simulink model "Last_Model_Interior_team"  (R2017b)
settings: Solver=VariableStepAuto  SolverName=FixedStepDiscrete  StartTime=0.0  StopTime=10  FixedStep=1e-6
PreLoadFcn:
  | %% Motor Parameters
  | Rs=6.9*10^-3;
  | Ld=220*10^-6;
  | Lq=265.4*10^-6;
  | Pm=87.78*10^-3;
  | P=4;
  | b=0.0019;
  | J=0.13;
  | f=50;
  | P_Rated=100000;
  | N_Rated=6320;
  | N_max=30000;
  | Tfl=P_Rated/(N_Rated*(2*pi/60));
  | Tl=0;
  | 
  | %% hardware impl
  | Vdc=340;
  | clocking=100;
  | fs=10000;
  | Ts=1/fs;
  | Irated=500;
  | Imax=500;
  | Id_MAX=-(Pm/Ld);
  | I_Limit=Irated;
  | I_fw=I_Limit;
  | Vmax=Vdc/sqrt(3);
  | update=2;
  | 
  | 
  | %% Inverter
  | Vdc=340;
  | deadtime=1e-6;
  | 
  | 
  | 
  | %% Tuning OF Id_Pole_Placment
  | zeta_Id=0.707;
  | Gamma_Id=0.9;
  | Wn_Id=(1/(1-Gamma_Id))*(Rs/Ld);
  | Kc_Id=(2*zeta_Id*Ld*Wn_Id)-Rs;
  | TAW_Id=((2*zeta_Id*Wn_Id*Ld)-Rs)/(Ld*Wn_Id*Wn_Id);
  | 
  | %% Tuning OF Iq_Pole_Placment
  | zeta_Iq=0.707;
  | Gamma_Iq=0.9;
  | Wn_Iq=(1/(1-Gamma_Iq))*(Rs/Lq);
  | Kc_Iq=(2*zeta_Iq*Lq*Wn_Iq)-Rs;
  | TAW_Iq=((2*zeta_Iq*Wn_Iq*Lq)-Rs)/(Lq*Wn_Iq*Wn_Iq);
  | 
  | 
  | 
  | %% Tuning of PI Using Symmetric Optimum For q phase
  | Tc=(1/fs)/update;
  | A=8;
  | Kp_SO_q=Lq/(A*(Tc)*1.5);
  | Ki_SO_q=1/((A^2)*1.5*Tc);
  | %% Tuning of PI Using Symmetric Optimum For d phase
  | Kp_SO_d=Ld/(A*(Tc)*1.5);
  | Ki_SO_d=1/((A^2)*1.5*Tc);
  | 
  | 
  | %% Tuning Of PI Using Magnetuide Optimum Q_phase
  | Ki_MO_q=Rs/Lq;
  | Kp_MO_q=Lq/(2*1.5*Tc);
  | %% Tuning Of PI Using Magnetuide Optimum D_phase
  | Ki_MO_d=Rs/Ld;
  | Kp_MO_d=Ld/(2*1.5*Tc);
  | %% Tuning Parameter
  | Kp_d=Kp_MO_d;
  | Ki_d=Ki_MO_d;
  | Kp_q=Kp_MO_q;
  | Ki_q=Ki_MO_q;
  | 
  | 
  | 
  | %% Tuning Speed Loop
  | Tcc=Tc*10;
  | M=4;
  | Kp_Speed=(8*J)/(3*M*9*Pm*Tcc);
  | Ki_Speed=M*M*Tcc;
InitFcn:
  | %% Motor Parameters
  | Rs=6.9*10^-3;
  | Ld=220*10^-6;
  | Lq=265.4*10^-6;
  | Pm=87.78*10^-3;
  | P=4;
  | b=0.0019;
  | J=0.13;
  | f=50;
  | P_Rated=100000;
  | N_Rated=6320;
  | N_max=30000;
  | Tfl=P_Rated/(N_Rated*(2*pi/60));
  | Tl=0;
  | 
  | %% hardware impl
  | Vdc=340;
  | clocking=100;
  | fs=10000;
  | Ts=1/fs;
  | Irated=500;
  | Imax=500;
  | Id_MAX=-(Pm/Ld);
  | I_Limit=Irated;
  | I_fw=I_Limit;
  | Vmax=Vdc/sqrt(3);
  | update=2;
  | 
  | %% Inverter
  | Vdc=340;
  | deadtime=1e-6;
  | 
  | 
  | 
  | %% Tuning OF Id_Pole_Placment
  | zeta_Id=0.707;
  | Gamma_Id=0.9;
  | Wn_Id=(1/(1-Gamma_Id))*(Rs/Ld);
  | Kc_Id=(2*zeta_Id*Ld*Wn_Id)-Rs;
  | TAW_Id=((2*zeta_Id*Wn_Id*Ld)-Rs)/(Ld*Wn_Id*Wn_Id);
  | 
  | %% Tuning OF Iq_Pole_Placment
  | zeta_Iq=0.707;
  | Gamma_Iq=0.9;
  | Wn_Iq=(1/(1-Gamma_Iq))*(Rs/Lq);
  | Kc_Iq=(2*zeta_Iq*Lq*Wn_Iq)-Rs;
  | TAW_Iq=((2*zeta_Iq*Wn_Iq*Lq)-Rs)/(Lq*Wn_Iq*Wn_Iq);
  | 
  | 
  | 
  | %% Tuning of PI Using Symmetric Optimum For q phase
  | Tc=(1/fs)/update;
  | A=8;
  | Kp_SO_q=Lq/(A*(Tc)*1.5);
  | Ki_SO_q=1/((A^2)*1.5*Tc);
  | %% Tuning of PI Using Symmetric Optimum For d phase
  | Kp_SO_d=Ld/(A*(Tc)*1.5);
  | Ki_SO_d=1/((A^2)*1.5*Tc);
  | 
  | 
  | %% Tuning Of PI Using Magnetuide Optimum Q_phase
  | Ki_MO_q=Rs/Lq;
  | Kp_MO_q=Lq/(2*1.5*Tc);
  | %% Tuning Of PI Using Magnetuide Optimum D_phase
  | Ki_MO_d=Rs/Ld;
  | Kp_MO_d=Ld/(2*1.5*Tc);
  | %% Tuning Parameter
  | Kp_d=Kp_MO_d;
  | Ki_d=Ki_MO_d;
  | Kp_q=Kp_MO_q;
  | Ki_q=Ki_MO_q;
  | 
  | 
  | 
  | %% Tuning Speed Loop
  | Tcc=Tc*10;
  | M=4;
  | Kp_Speed=(8*J)/(3*M*9*Pm*Tcc);
  | Ki_Speed=M*M*Tcc;
undefined symbols (not defined in the file): DiscIntNeverNeededParam, magnitude
libraries: simulink x81, powerlib x14
(part 1 of 4)
CloseFcn:
  | clc;
  | clear;
settings Model: PauseTimes=0.2  Creator=oem  LastModifiedBy=Abdo
settings SolverCC: ZeroCrossAlgorithm=Adaptive
settings DataIOCC: SaveOutput=off  DSMLogging=off  SaveTime=off
settings OptimizationCC: UseDivisionForNetSlopeComputation=on  UseFloatMulNetSlope=on  DefaultUnderspecifiedDataType=single  EnhancedBackFolding=on  BooleansAsBitfields=on  PassReuseOutputArgsAs=Individual arguments  StateBitsets=on  DataBitsets=on  ZeroExternalMemoryAtStartup=off  ZeroInternalMemoryAtStartup=off  NoFixptDivByZeroProtection=on  EfficientFloat2IntCast=on  LifeSpan=1  MaxStackSize=64  OptimizeBlockOrder=speed  DifferentSizesBufferReuse=on
settings DebuggingCC: IgnoredZcDiagnostic=none  ParameterTunabilityLossMsg=error  UnconnectedInputMsg=none  UnconnectedOutputMsg=none  UnconnectedLineMsg=none
settings HardwareCC: ProdBitPerPointer=32  ProdBitPerSizeT=32  ProdBitPerPtrDiffT=32  ProdLargestAtomicFloat=None  ProdWordSize=32  ProdHWDeviceType=Atmel->AVR (32-bit)
settings ModelReferenceCC: EnableRefExpFcnMdlSchedulingChecks=off
settings SFSimCC: SimUseLocalCustomCode=on  MATLABDynamicMemAlloc=off
settings RTWCC: SystemTargetFile=ert.tlc  TemplateMakefile=ert_default_tmf  RTWUseLocalCustomCode=on  Toolchain=Texas Instruments Code Composer Studio (C2000)
settings CodeAppCC: ForceParamTrailComments=on  IgnoreCustomStorageClasses=off  OperatorAnnotations=on  SimulinkDataObjDesc=on  SFDataObjDesc=on  CustomSymbolStrGlobalVar=rt$N$M  CustomSymbolStrType=$N$M  CustomSymbolStrFcn=$N$M$F  CustomSymbolStrMacro=$N$M  InsertBlockDesc=on
settings ERTTargetCC: IncludeMdlTerminateFcn=off  CombineSignalStateStructs=on  CodeInterfacePackaging=Reusable function  SupportComplex=off  SupportNonInlinedSFcns=on  ExtModeStaticAlloc=on  ERTCustomFileTemplate=example_file_process.tlc  ERTFilePackagingFormat=CompactWithDataFile  MemSecPackage=Simulink

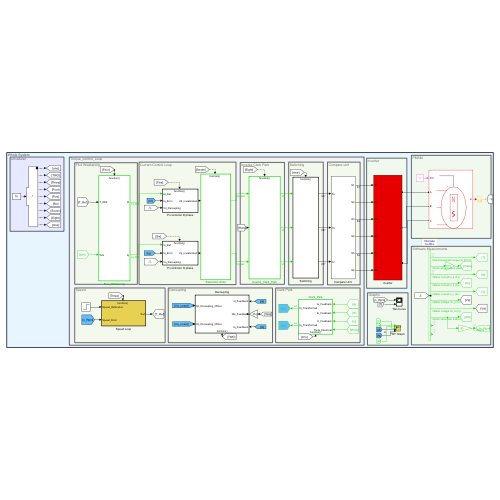
[thumbnail: Simulink's stored preview of the top-level diagram]
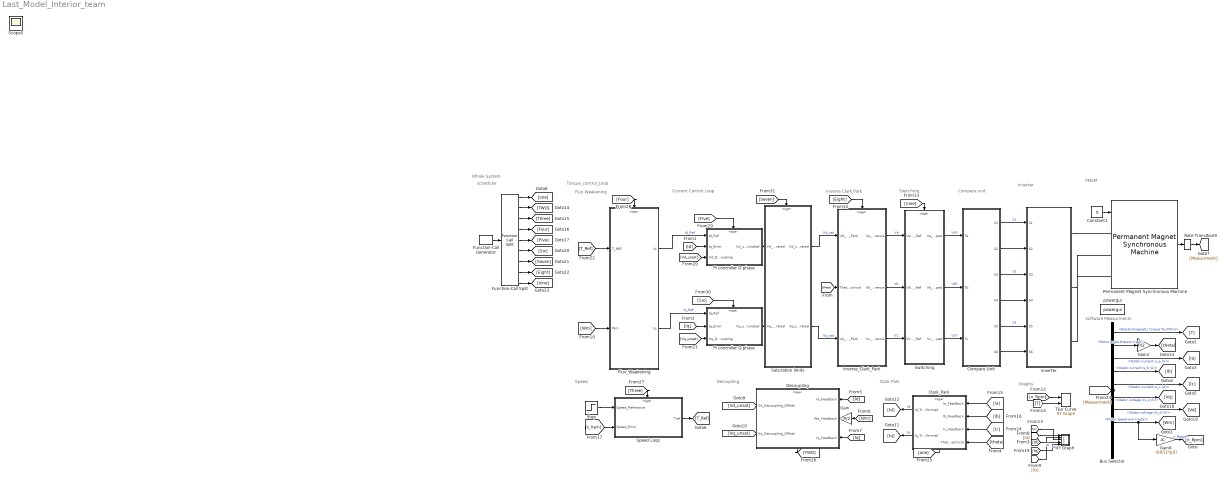
== system Last_Model_Interior_team ==
  note: schedular
  note: Software Measurments
  note: Torque_control_Loop
  note: Graphs
  note: Clark Park
  note: Flux Weakening
  note: Inverter
  note: Whole System
  note: Decoupling
  note: Inverse Clark Park
  note: Current Control Loop
  note: PMSM
  note: Switching
  note: Speed
  note: Compare unit
  Bus Selector : BusSelector  OutputSignals=Electromagnetic torque Te (N*m),Rotor angle thetam (rad),Stator current is_a (A),Stator current is_b (A),Stator current is_c (A),Stator voltage Vs_q (V),Stator voltage Vs_d (V),Rotor speed wm (rad/s),Stator current is_q (A),Stator current is_d (A)
  Clark_Park : Subsystem  TreatAsAtomicUnit=on
  "Compare Unit " : Subsystem
  Constant1 : Constant  Value=0
  Decoupling : Subsystem  TreatAsAtomicUnit=on
  Flux_Weakening : Subsystem
  Function-Call Generator : simulink/Ports & Subsystems/Function-Call Generator  sample_time=Tc  numberOfIterations=1
  Function-Call Split : FunctionCallSplit  IconShape=distinctive  NumOutputPorts=9  OutputPortLayout=default
  Gain : Gain  Gain=P/2
  Gain2 : Gain  Gain=P/2
  Gain8 : Gain  Gain=(60/(2*pi))
  Inverse_Clark_Park : Subsystem
  Permanent Magnet Synchronous Machine : powerlib/Machines/Permanent Magnet Synchronous Machine  NbPhases=3  FluxDistribution=Sinusoidal  RotorType=Salient-pole  MechanicalLoad=Torque Tm  PresetModel=No  ShowDetailedParameters=on  MeasurementBus=off  Resistance=Rs  Inductance=8.5e-3  dqInductances=[Ld Lq]  La=Ld  MachineConstant=Flux linkage established by magnets (V.s)  Flux=Pm  VoltageCst=31.8431  TorqueCst=0.26334  Flat=120  Mechanical=[J b P/2 0]  PolePairs=4  InitialConditions=[0,0, 0,0]  InitialConditions5ph=[0 0 0 0 0 0]  RefAngle=Aligned with phase A axis (original Park)  IterativeDiscreteModel=Trapezoidal non iterative  TsBlock=-1  TsPowergui=0
  Pi controller D phase : Subsystem
  Pi controller Q phase : Subsystem
  Rate Transition9 : RateTransition  OutPortSampleTime=Tc
  Saturation limits : Subsystem
  Speed Loop : Subsystem
  Step : Step  Time=0.000000001  After=5000  SampleTime=0
  Switching : Subsystem  SystemSampleTime=1e-4
  T&n Curve : simulink/Sinks/XY Graph  xmin=-1  xmax=1  ymin=-1  ymax=1  st=-1
  XY Graph : Subsystem  Description=Replaced Block  mask(Replaced Block){}
      mask help: This block has been replaced with an empty subsystem because it used functionality that is unavailable in Simulink R2017b.
      mask Display: fprintf('Replaced: %s\n','Record')
  inverter : Subsystem
  powergui : powerlib/powergui  Priority=1  SimulationMode=Discrete  SampleTime=1e-6  frequency=60  Iterations=50  frequencyindice=0  Pbase=100e6  ErrMax=1e-4  UnitsV=kV  UnitsW=MW  buscounter=0  FunctionMessages=off  echomessages=off  EnableUseOfTLC=off  CurrentSourceSwitches=off  DisableSnubberDevices=off  DisableRonSwitches=off  DisableVfSwitches=off  DisplayEquations=off  AutomaticDiscreteSolvers=off  SolverType=Tustin/Backward Euler (TBE)  Interpol=off  ExternalGateDelay=off  methode=off  Ts=100  x0status=blocks  SPID=on  SwTol=0  HookPort=off  NonlinearTolerance=1e-4  nMaxIteration=100  ContinueOnMaxIteration=off  RestoreLinks=warning  ResistiveCurrentMeasurement=off  Frange=[0:2:500]  Ylog=off  Xlog=on  ShowGrid=off  save=off  variable=ZData  structure=0  ZoomFFT=off  StartTime=0.0  cycles=1  DisplayStyle=1  fundamental=60  FreqAxis=off  MaxFrequency=1000  frequencyindicesteady=1  RmsSteady=1  display=off
  Scope5 : Scope
  wires:
  [Id] -> Decoupling/1(Id_Feedback)
  [Iq] -> Decoupling/3(Iq_Feedback)
  Decoupling/1(Vd_Decoupling_Offset) -> [Vd_unsat]
  Decoupling/2(Vq_Decoupling_Offset) -> [Vq_unsat]
  [Wm] -> Gain/1
  Gain/1 -> Decoupling/2(We_Feedback)
  [theta] -> Inverse_Clark_Park/2(Theta_Electrical)
  [n_Rpm] -> T&n Curve/1
  [T] -> T&n Curve/2
  [Ia] -> Clark_Park/1(Ia_Feedback)
  [Ib] -> Clark_Park/2(Ib_Feedback)
  [theta] -> Clark_Park/4(Theta_Electrical)
  Clark_Park/1(Id_Transformed) -> [Id]  "Id"
  Clark_Park/2(Iq_Transformed) -> [Iq]  "Iq"
  [Iq] -> XY Graph/5(In5)  "iq"
  [Id] -> XY Graph/4(In4)  "id"
  Saturation limits/1(Vd_saturated) -> Inverse_Clark_Park/1(Vd_Refrence_To_Inverse_Clark_Park)  "Vd_sat"
  Saturation limits/2(Vq_saturated) -> Inverse_Clark_Park/3(Vq_Refrence_To_Inverse_Clark_Park)  "Vq_sat"
  Bus Selector/1 -> [T]  "<Electromagnetic torque Te (N*m)>"
  Bus Selector/2 -> Gain2/1  "<Rotor angle thetam (rad)>"
  Bus Selector/4 -> [Ib]  "<Stator current is_b (A)>"
  Permanent Magnet Synchronous Machine/1 -> Rate Transition9/1
  Rate Transition9/1 -> [Measurment]
  Bus Selector/3 -> [Ia]  "<Stator current is_a (A)>"
  Bus Selector/5 -> [Ic]  "<Stator current is_c (A)>"
  Bus Selector/8 -> [Wm], Gain8/1  "<Rotor speed wm (rad/s)>"
  Gain8/1 -> [n_Rpm]  "n_Rpppm"
  [Wm] -> Flux_Weakening/2(Wm)
  Bus Selector/6 -> [Vq]  "<Stator voltage Vs_q (V)>"
  Bus Selector/7 -> [Vd]  "<Stator voltage Vs_d (V)>"
  Constant1/1 -> Permanent Magnet Synchronous Machine/1
  [Ia] -> XY Graph/1(In1)
  [Ib] -> XY Graph/2(In2)
  [Ic] -> XY Graph/3(In3)
  [Measurment] -> Bus Selector/1
  Inverse_Clark_Park/1(Va_Sin_Wave_Reference) -> Switching/1(Va_Sin_Ref)  "Va"
  Inverse_Clark_Park/2(Vb_Sin_Wave_Reference) -> Switching/2(Vb_Sin_Ref)  "Vb"
  Inverse_Clark_Park/3(Vc_Sin_Wave_Reference) -> Switching/3(Vc_Sin_Ref)  "VC"
  [Ic] -> Clark_Park/3(Ic_Feedback)
  [T_Ref] -> Flux_Weakening/1(T_REF)
  Switching/1(Va_Bus_Clamped) -> "Compare Unit "/1(Ta)  "VA*"
  Switching/2(Vb_Bus_Clamped) -> "Compare Unit "/2(Tb)  "VB*"
  Switching/3(Vc_Bus_Clamped) -> "Compare Unit "/3(Tc)  "VC*"
  "Compare Unit "/1(S1) -> inverter/1(S1)  "S1"
  "Compare Unit "/2(S2) -> inverter/2(S2)
  "Compare Unit "/4(S4) -> inverter/4(S4)
  "Compare Unit "/6(S6) -> inverter/6(S6)
  "Compare Unit "/3(S3) -> inverter/3(S3)  "S2"
  "Compare Unit "/5(S5) -> inverter/5(S5)  "S3"
  Step/1 -> Speed Loop/1(Speed_Referance)
  [n_Rpm] -> Speed Loop/2(Speed_Error)
  Speed Loop/1(Tref) -> [T_Ref]
  Flux_Weakening/1(Id) -> Pi controller D phase/1(Id_Ref)  "Id_Ref"
  [Id] -> Pi controller D phase/2(Iq_Error)
  [Vd_unsat] -> Pi controller D phase/3(Vd_Decoupling)
  Pi controller D phase/1(Vd_unsaturated) -> Saturation limits/1(Vd_unsaturated)
  Flux_Weakening/2(Iq) -> Pi controller Q phase/1(Iq_Ref)  "Iq_Ref"
  [Iq] -> Pi controller Q phase/2(Iq_Error)
  [Vq_unsat] -> Pi controller Q phase/3(Vq_Decoupling)
  Pi controller Q phase/1(Vq_unsaturated) -> Saturation limits/2(Vq_unsaturated)
  Function-Call Generator/1 -> Function-Call Split/1
  [one] -> Clark_Park/Trigger
  Function-Call Split/1 -> [one]
  Function-Call Split/2 -> [TWO]
  Function-Call Split/3 -> [Three]
  Function-Call Split/4 -> [Four]
  Function-Call Split/5 -> [Five]
  Function-Call Split/6 -> [Six]
  Function-Call Split/7 -> [Seven]
  [TWO] -> Decoupling/Trigger
  [Four] -> Flux_Weakening/Trigger
  [Five] -> Pi controller D phase/Trigger
  [Six] -> Pi controller Q phase/Trigger
  [Seven] -> Saturation limits/Trigger
  Function-Call Split/8 -> [Eight]
  Function-Call Split/9 -> [nine]
  [Eight] -> Inverse_Clark_Park/Trigger
  [nine] -> Switching/Trigger
  Gain2/1 -> [theta]
  [Three] -> Speed Loop/Trigger
  connections:
  inverter/RConn1 -- Permanent Magnet Synchronous Machine/LConn1
  inverter/RConn2 -- Permanent Magnet Synchronous Machine/LConn2
  inverter/RConn3 -- Permanent Magnet Synchronous Machine/LConn3

== system Last_Model_Interior_team/Clark_Park ==
  Ia_Feedback : Inport
  Ib_Feedback : Inport  Port=2
  Ic_Feedback : Inport  Port=3
  Theta_Electrical : Inport  Port=4
  function : TriggerPort  TriggerType=function-call  VariantControl=(inherit)
  Constant : Constant  Value=(2*pi)/3
  Constant1 : Constant  Value=(4*pi)/3
  Constant2 : Constant  Value=(2*pi)/3
  Constant3 : Constant  Value=(4*pi)/3
  Cos2 : Trigonometry  Operator=cos
  Cos3 : Trigonometry  Operator=cos
  Cos4 : Trigonometry  Operator=cos
  Cos5 : Trigonometry
  Cos6 : Trigonometry
  Cos7 : Trigonometry
  Gain8 : Gain  Gain=2/3
  Gain9 : Gain  Gain=-2/3
  Product{4..9} (6 alike) : Product
  Sum{4..5,7..8} (4 alike) : Sum  Inputs=-+
  Sum6 : Sum  Inputs=+++
  Sum9 : Sum  Inputs=+++
  Id_Transformed : Outport
  Iq_Transformed : Outport  Port=2
  wires:
  Theta_Electrical/1 -> Cos5/1, Sum7/2, Sum8/2, Sum4/2, Cos2/1, Sum5/2
  Sum4/1 -> Cos3/1
  Constant/1 -> Sum4/1
  Constant1/1 -> Sum5/1
  Sum5/1 -> Cos4/1
  Cos2/1 -> Product4/2
  Cos3/1 -> Product5/1
  Cos4/1 -> Product6/1
  Product5/1 -> Sum6/2
  Product4/1 -> Sum6/1
  Product6/1 -> Sum6/3
  Sum6/1 -> Gain8/1
  Gain8/1 -> Id_Transformed/1
  Sum8/1 -> Cos7/1
  Gain9/1 -> Iq_Transformed/1
  Product8/1 -> Sum9/2
  Product9/1 -> Sum9/3
  Product7/1 -> Sum9/1
  Constant3/1 -> Sum8/1
  Cos7/1 -> Product9/1
  Constant2/1 -> Sum7/1
  Sum7/1 -> Cos6/1
  Cos6/1 -> Product8/1
  Sum9/1 -> Gain9/1
  Cos5/1 -> Product7/2
  Ia_Feedback/1 -> [a]
  Ib_Feedback/1 -> [b]
  Ic_Feedback/1 -> [c]
  [a] -> Product4/1
  [b] -> Product5/2
  [c] -> Product6/2
  [a] -> Product7/1
  [b] -> Product8/2
  [c] -> Product9/2

== system Last_Model_Interior_team/Compare Unit  ==
  Ta : Inport
  Tb : Inport  Port=2
  Tc : Inport  Port=3
  AND{,1..5} (6 alike) : Logic  IconShape=distinctive  AllPortsSameDT=off  OutDataTypeStr=boolean
  Add : Sum  Inputs=+-
  Carrier Wave1 : simulink/Sources/Repeating Sequence  rep_seq_t=[0 0.5 1]/((fs))  rep_seq_y=[0 100 0]
  NOT : Logic  Operator=NOT  IconShape=distinctive  AllPortsSameDT=off  OutDataTypeStr=boolean
  NOT1 : Logic  Operator=NOT  IconShape=distinctive  AllPortsSameDT=off  OutDataTypeStr=boolean
  NOT3 : Logic  Operator=NOT  IconShape=distinctive  AllPortsSameDT=off  OutDataTypeStr=boolean
  Relational Operator : RelationalOperator  OutDataTypeStr=boolean  RndMeth=Ceiling
  Relational Operator1 : RelationalOperator  OutDataTypeStr=boolean  RndMeth=Ceiling
  Relational Operator2 : RelationalOperator  OutDataTypeStr=boolean  RndMeth=Ceiling
  Scope : Scope  NumInputPorts=2
  Scope1 : Scope  NumInputPorts=2
  Scope2 : Scope
  Unit Delay{,1..5} (6 alike) : UnitDelay  SampleTime=deadtime  HasFrameUpgradeWarning=on
  S1 : Outport  VectorParamsAs1DForOutWhenUnconnected=off
  S2 : Outport  Port=2  VectorParamsAs1DForOutWhenUnconnected=off
  S3 : Outport  Port=3  VectorParamsAs1DForOutWhenUnconnected=off
  S4 : Outport  Port=4  VectorParamsAs1DForOutWhenUnconnected=off
  S5 : Outport  Port=5  VectorParamsAs1DForOutWhenUnconnected=off
  S6 : Outport  Port=6  VectorParamsAs1DForOutWhenUnconnected=off
  wires:
  Ta/1 -> Relational Operator/1, Scope1/1
  Tc/1 -> Relational Operator2/1
  Tb/1 -> Relational Operator1/1
  Relational Operator/1 -> Add/1, NOT/1, Unit Delay/1, AND/1
  Unit Delay/1 -> AND/2
  AND/1 -> Scope/1, S1/1, Add/2
  NOT/1 -> Unit Delay1/1, AND1/1
  Unit Delay1/1 -> AND1/2
  AND1/1 -> S2/1, Scope/2
  Unit Delay3/1 -> AND3/2
  NOT3/1 -> Unit Delay3/1, AND3/1
  Unit Delay2/1 -> AND2/2
  Relational Operator1/1 -> AND2/1, Unit Delay2/1, NOT3/1
  AND2/1 -> S3/1
  AND3/1 -> S4/1
  Relational Operator2/1 -> NOT1/1, Unit Delay4/1, AND4/1
  Unit Delay4/1 -> AND4/2
  NOT1/1 -> Unit Delay5/1, AND5/1
  Unit Delay5/1 -> AND5/2
  AND4/1 -> S5/1
  AND5/1 -> S6/1
  Add/1 -> Scope2/1
  Carrier Wave1/1 -> Scope1/2, Relational Operator/2, Relational Operator2/2, Relational Operator1/2  "Carrier_Wave"

== system Last_Model_Interior_team/Decoupling ==
  Id_Feedback : Inport
  We_Feedback : Inport  Port=2
  Iq_Feedback : Inport  Port=3
  function : TriggerPort  TriggerType=function-call  VariantControl=(inherit)
  Add : Sum
  Constant : Constant  Value=Ld
  Constant1 : Constant  Value=Lq
  Constant2 : Constant  Value=Pm
  Product : Product
  Product1 : Product
  Product2 : Product  Inputs=3
  Vd_Decoupling_Offset : Outport
  Vq_Decoupling_Offset : Outport  Port=2
  wires:
  Constant1/1 -> Product2/1
  Iq_Feedback/1 -> Product2/3
  Product2/1 -> Vd_Decoupling_Offset/1
  Id_Feedback/1 -> Product/2
  Product/1 -> Add/1
  Constant2/1 -> Add/2
  Product1/1 -> Vq_Decoupling_Offset/1
  We_Feedback/1 -> Product1/2, Product2/2
  Add/1 -> Product1/1
  Constant/1 -> Product/1

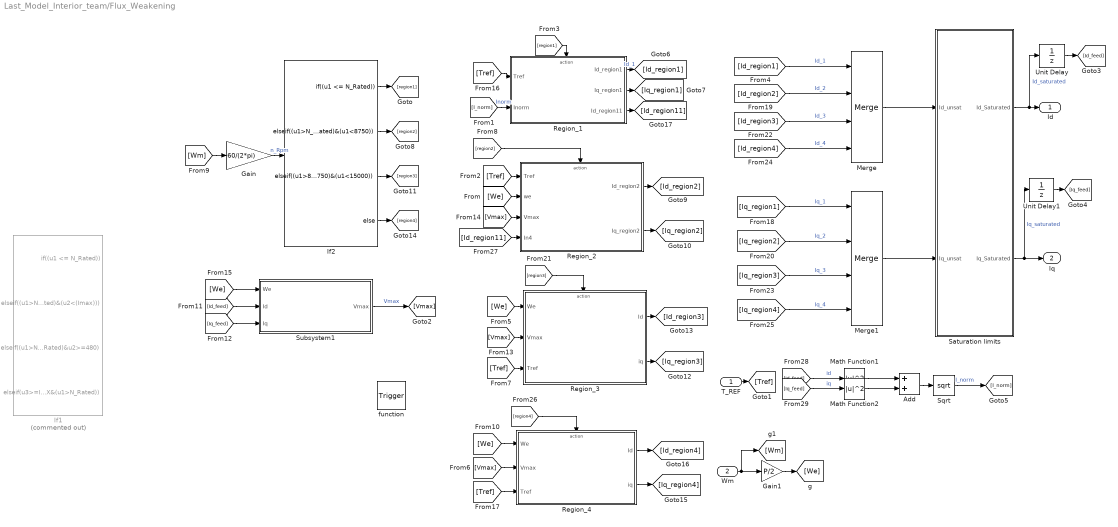
== system Last_Model_Interior_team/Flux_Weakening ==
  T_REF : Inport
  Wm : Inport  Port=2
  function : TriggerPort  TriggerType=function-call  VariantControl=(inherit)
  Add : Sum
  Gain : Gain  Gain=60/(2*pi)
  Gain1 : Gain  Gain=P/2
  If1 : If  Commented=on  NumInputs=3  IfExpression=(u1 <= N_Rated)  ElseIfExpressions=(u1>N_Rated)&(u2<(Imax)),(u1>N_Rated)&u2>=480,u3>=Id_MAX&(u1>N_Rated)  ShowElse=off
  If2 : If  IfExpression=(u1 <= N_Rated)  ElseIfExpressions=(u1>N_Rated)&(u1<8750),(u1>8750)&(u1<15000)
  Math Function1 : Math  Operator=magnitude^2  OutputSignalType=real  SaturateOnIntegerOverflow=on
  Math Function2 : Math  Operator=magnitude^2  OutputSignalType=real  SaturateOnIntegerOverflow=on
  Merge : Merge  Inputs=4
  Merge1 : Merge  Inputs=4
  Region_1 : Subsystem  TreatAsAtomicUnit=on
  Region_2 : Subsystem  TreatAsAtomicUnit=on
  Region_3 : Subsystem  TreatAsAtomicUnit=on
  Region_4 : Subsystem  TreatAsAtomicUnit=on
  Saturation limits : Subsystem
  Sqrt : Sqrt  OutputSignalType=real  SaturateOnIntegerOverflow=on
  Subsystem1 : Subsystem
  Unit Delay : UnitDelay  SampleTime=-1  HasFrameUpgradeWarning=on
  Unit Delay1 : UnitDelay  SampleTime=-1  HasFrameUpgradeWarning=on
  Id : Outport
  Iq : Outport  Port=2
  wires:
  [Tref] -> Region_1/1(Tref)
  Gain/1 -> If2/1  "n_Rpm"
  Wm/1 -> Gain1/1, [Wm]
  T_REF/1 -> [Tref]
  Gain1/1 -> [We]
  [Tref] -> Region_2/1(Tref)
  [We] -> Region_2/2(we)
  Sqrt/1 -> [I_norm]  "I_norm"
  [Id_feed] -> Math Function1/1  "id"
  Math Function1/1 -> Add/1
  Math Function2/1 -> Add/2
  Add/1 -> Sqrt/1
  [We] -> Region_3/1(We)
  [Iq_feed] -> Math Function2/1  "iq"
  [Id_feed] -> Subsystem1/2(Id)
  [We] -> Subsystem1/1(We)
  [Iq_feed] -> Subsystem1/3(Iq)
  Subsystem1/1(Vmax) -> [Vmax]  "Vmax"
  [Wm] -> Gain/1
  [Vmax] -> Region_2/3(Vmax)
  [Vmax] -> Region_3/2(Vmax)
  [I_norm] -> Region_1/2(Inorm)  "Inorm"
  [Vmax] -> Region_4/2(Vmax)
  [We] -> Region_4/1(We)
  Merge/1 -> Saturation limits/1(Id_unsat)
  Merge1/1 -> Saturation limits/2(Iq_unsat)
  Saturation limits/1(Id_Saturated) -> Unit Delay/1, Id/1  "Id_saturated"
  Saturation limits/2(Iq_Saturated) -> Iq/1, Unit Delay1/1  "Iq_saturated"
  [region1] -> Region_1/Action
  Region_1/1(Id_region1) -> [Id_region1]  "Id_1"
  Region_1/2(Iq_region1) -> [Iq_region1]
  [Id_region1] -> Merge/1  "Id_1"
  [Iq_region1] -> Merge1/1  "Iq_1"
  [region2] -> Region_2/Action
  Region_2/1(Id_region2) -> [Id_region2]
  Region_2/2(Iq_region2) -> [Iq_region2]
  [Id_region2] -> Merge/2  "Id_2"
  [Iq_region2] -> Merge1/2  "Iq_2"
  [region3] -> Region_3/Action
  Region_3/1(Id) -> [Id_region3]
  Region_3/2(iq) -> [Iq_region3]
  [Id_region3] -> Merge/3  "Id_3"
  [Iq_region3] -> Merge1/3  "Iq_3"
  Region_4/1(Id) -> [Id_region4]
  Region_4/2(iq) -> [Iq_region4]
  [Id_region4] -> Merge/4  "Id_4"
  [Iq_region4] -> Merge1/4  "Iq_4"
  [region4] -> Region_4/Action
  [Id_region11] -> Region_2/4(In4)
  Region_1/3(Id_region11) -> [Id_region11]
  If2/1 -> [region1]
  If2/2 -> [region2]
  If2/3 -> [region3]
  If2/4 -> [region4]
  [Tref] -> Region_3/3(Tref)
  [Tref] -> Region_4/3(Tref)
  Unit Delay/1 -> [Id_feed]
  Unit Delay1/1 -> [Iq_feed]

== system Last_Model_Interior_team/Inverse_Clark_Park ==
  Vd_Refrence_To_Inverse_Clark_Park : Inport
  Theta_Electrical : Inport  Port=2
  Vq_Refrence_To_Inverse_Clark_Park : Inport  Port=3
  function : TriggerPort  TriggerType=function-call  VariantControl=(inherit)
  Constant{1..4} (4 alike) : Constant  Value=(2*pi)/3
  Cos1 : Trigonometry  Operator=cos
  Cos2 : Trigonometry  Operator=cos
  Cos3 : Trigonometry
  Cos4 : Trigonometry
  Cos5 : Trigonometry  Operator=cos
  Cos6 : Trigonometry
  Gain : Gain  Gain=-1
  Gain1 : Gain  Gain=-1
  Gain2 : Gain  Gain=-1
  Product{1..2,4..5,7..8} (6 alike) : Product
  Sum{1..3,7,10} (5 alike) : Sum
  Sum5 : Sum  Inputs=-+
  Sum8 : Sum  Inputs=-+
  Va_Sin_Wave_Reference : Outport
  Vb_Sin_Wave_Reference : Outport  Port=2
  Vc_Sin_Wave_Reference : Outport  Port=3
  wires:
  Product4/1 -> Sum7/1
  Cos5/1 -> Product7/2
  Sum8/1 -> Cos6/1
  Product7/1 -> Sum10/1
  Cos6/1 -> Gain1/1
  Cos2/1 -> Product4/2
  Product8/1 -> Sum10/2
  Sum7/1 -> Va_Sin_Wave_Reference/1
  Sum10/1 -> Vb_Sin_Wave_Reference/1
  [d] -> Product7/1
  [d] -> Product4/1
  Constant2/1 -> Sum8/1
  [q] -> Product8/2
  Vd_Refrence_To_Inverse_Clark_Park/1 -> [d]
  Vq_Refrence_To_Inverse_Clark_Park/1 -> [q]
  [q] -> Product5/1
  Cos3/1 -> Gain/1
  Product5/1 -> Sum7/2
  Gain/1 -> Product5/2
  Constant1/1 -> Sum5/1
  Sum5/1 -> Cos5/1
  Gain1/1 -> Product8/1
  Gain2/1 -> Product2/1
  Sum2/1 -> Cos1/1
  Constant4/1 -> Sum2/1
  Theta_Electrical/1 -> Sum3/2, Sum2/2, Sum8/2, Sum5/2, Cos2/1, Cos3/1
  [q] -> Product2/2
  Constant3/1 -> Sum3/1
  [d] -> Product1/1
  Sum1/1 -> Vc_Sin_Wave_Reference/1
  Product2/1 -> Sum1/2
  Cos4/1 -> Gain2/1
  Product1/1 -> Sum1/1
  Sum3/1 -> Cos4/1
  Cos1/1 -> Product1/2

== system Last_Model_Interior_team/Pi controller D phase ==
  Id_Ref : Inport
  Iq_Error : Inport  Port=2
  Vd_Decoupling : Inport  Port=3
  function : TriggerPort  TriggerType=function-call  VariantControl=(inherit)
  Pi D Phase : Subsystem  TreatAsAtomicUnit=on
  Sum : Sum  Inputs=|+-
  Sum4 : Sum  Inputs=|+-
  Vd_unsaturated : Outport
  wires:
  Sum/1 -> Pi D Phase/1(Id*)  "error_Id"
  Iq_Error/1 -> Sum/2
  Pi D Phase/1(Vd) -> Sum4/1
  Id_Ref/1 -> Sum/1
  Sum4/1 -> Vd_unsaturated/1  "Vd_unsat"
  Vd_Decoupling/1 -> Sum4/2

== system Last_Model_Interior_team/Pi controller Q phase ==
  Iq_Ref : Inport
  Iq_Error : Inport  Port=2
  Vq_Decoupling : Inport  Port=3
  function : TriggerPort  TriggerType=function-call  VariantControl=(inherit)
  PI controller : Subsystem  TreatAsAtomicUnit=on
  Sum1 : Sum  Inputs=|+-
  Sum5 : Sum  Inputs=|++
  Vq_unsaturated : Outport
  wires:
  PI controller/1(Vq) -> Sum5/1
  Sum5/1 -> Vq_unsaturated/1  "Vq_unsat"
  Sum1/1 -> PI controller/1(Iq*)  "error_iq"
  Iq_Ref/1 -> Sum1/1
  Iq_Error/1 -> Sum1/2
  Vq_Decoupling/1 -> Sum5/2

== system Last_Model_Interior_team/Saturation limits ==
  Vd_unsaturated : Inport
  Vq_unsaturated : Inport  Port=2
  function : TriggerPort  TriggerType=function-call  VariantControl=(inherit)
  Abs : Abs
  Abs1 : Abs
  Add : Sum
  Constant : Constant  Value=Vmax
  Constant2 : Constant  Value=Vmax
  Divide : Product  Inputs=**/
  Divide1 : Product  Inputs=**/
  Math Function : Math  Operator=magnitude^2  SaturateOnIntegerOverflow=on
  Math Function1 : Math  Operator=magnitude^2  SaturateOnIntegerOverflow=on
  Multiply : Gain  Gain=-1
  Multiply1 : Gain  Gain=-1
  Saturation Dynamic : simulink/Discontinuities/Saturation Dynamic  OutMin=[]  OutMax=[]  OutDataTypeStr=Inherit: Same as second input  OutDataType=fixdt(1, 16)  OutScaling=2^-10  DoSatur=off
  Saturation Dynamic1 : simulink/Discontinuities/Saturation Dynamic  OutMin=[]  OutMax=[]  OutDataTypeStr=Inherit: Same as second input  OutDataType=fixdt(1, 16)  OutScaling=2^-10  DoSatur=off
  Sqrt : Sqrt  SaturateOnIntegerOverflow=on
  Zero detection : Subsystem
  Vd_saturated : Outport
  Vq_saturated : Outport  Port=2
  wires:
  Vd_unsaturated/1 -> [Vd_unsat], Abs1/1, Math Function1/1
  Math Function/1 -> Add/1
  Math Function1/1 -> Add/2
  Add/1 -> Sqrt/1
  Sqrt/1 -> Zero detection/1(In1)
  Zero detection/1(Out1) -> Divide1/3, Divide/3  "Vs_unsat"
  Vq_unsaturated/1 -> [Vq_unsat], Abs/1, Math Function/1
  Abs/1 -> Divide/2
  Constant/1 -> Divide/1
  Constant2/1 -> Divide1/1
  Abs1/1 -> Divide1/2
  Divide/1 -> Saturation Dynamic/1, Multiply/1
  [Vq_unsat] -> Saturation Dynamic/2
  Multiply/1 -> Saturation Dynamic/3
  [Vd_unsat] -> Saturation Dynamic1/2
  Divide1/1 -> Multiply1/1, Saturation Dynamic1/1
  Multiply1/1 -> Saturation Dynamic1/3
  Saturation Dynamic/1 -> Vq_saturated/1
  Saturation Dynamic1/1 -> Vd_saturated/1

== system Last_Model_Interior_team/Speed Loop ==
  Speed_Referance : Inport
  Speed_Error : Inport  Port=2
  function : TriggerPort  TriggerType=function-call  VariantControl=(inherit)
  Sum2 : Sum  Inputs=|+-
  speed_controller : Subsystem  TreatAsAtomicUnit=on
  Tref : Outport
  wires:
  Speed_Referance/1 -> Sum2/1
  Sum2/1 -> speed_controller/1(ref_speed)  "error_n"
  Speed_Error/1 -> Sum2/2
  speed_controller/1(T_ref) -> Tref/1

== system Last_Model_Interior_team/Switching ==
  Va_Sin_Ref : Inport
  Vb_Sin_Ref : Inport  Port=2
  Vc_Sin_Ref : Inport  Port=3
  function : TriggerPort  TriggerType=function-call  VariantControl=(inherit)
  +120_deg_Dpwm : Subsystem  Commented=on
  -120_deg_Dpwm : Subsystem  Commented=on
  30_deg_Dpwm : Subsystem  Commented=on
  60deg_+30_shifted : Subsystem  Commented=on
  60deg_-30_shifted : Subsystem  Commented=on
  60deg_DPWM : Subsystem
  SVpwm : Subsystem  Commented=on
  Scope : Scope  Commented=on  NumInputPorts=3
  Va_Bus_Clamped : Outport
  Vb_Bus_Clamped : Outport  Port=2
  Vc_Bus_Clamped : Outport  Port=3
  wires:
  ? -> +120_deg_Dpwm/2(Vb)
  ? -> +120_deg_Dpwm/3(Vc)
  ? -> +120_deg_Dpwm/1(Va)
  +120_deg_Dpwm/1(Va*) -> ?
  +120_deg_Dpwm/2(Vb*) -> ?
  +120_deg_Dpwm/3(Vc*) -> ?
  ? -> 30_deg_Dpwm/1(Va), Scope/1
  ? -> 30_deg_Dpwm/2(Vb), Scope/2
  ? -> 30_deg_Dpwm/3(Vc), Scope/3
  30_deg_Dpwm/3(Vc*) -> ?
  30_deg_Dpwm/2(Vb*) -> ?
  30_deg_Dpwm/1(Va*) -> ?
  Va_Sin_Ref/1 -> 60deg_DPWM/1(Va)
  Vb_Sin_Ref/1 -> 60deg_DPWM/2(Vb)
  Vc_Sin_Ref/1 -> 60deg_DPWM/3(Vc)
  60deg_DPWM/1(Va_Bus_Clamped) -> Va_Bus_Clamped/1
  60deg_DPWM/2(Vb_Bus_Clamped) -> Vb_Bus_Clamped/1
  60deg_DPWM/3(Vc_Bus_Clamped) -> Vc_Bus_Clamped/1

== system Last_Model_Interior_team/XY Graph ==
  In1 : Inport
  In2 : Inport  Port=2
  In3 : Inport  Port=3
  In4 : Inport  Port=4
  In5 : Inport  Port=5
  Terminator{1..5} (5 alike) : Terminator
  wires:
  In5/1 -> Terminator5/1
  In4/1 -> Terminator4/1
  In3/1 -> Terminator3/1
  In2/1 -> Terminator2/1
  In1/1 -> Terminator1/1

== system Last_Model_Interior_team/inverter ==
  S1 : Inport
  S2 : Inport  Port=2
  S3 : Inport  Port=3
  S4 : Inport  Port=4
  S5 : Inport  Port=5
  S6 : Inport  Port=6
  Current Measurement : powerlib/Measurements/Current Measurement  PhasorSimulation=off  OutputType=Complex  PSBequivalent=0
  DC Voltage Source : powerlib/Electrical Sources/DC Voltage Source  Amplitude=Vdc  Measurements=None
  IGBT/Diode : powerlib/Power Electronics/IGBT//Diode  Ron=1e-3  Rs=1e5  Cs=10e2  Measurements=on
  IGBT/Diode{1..5} (5 alike) : powerlib/Power Electronics/IGBT//Diode  Ron=1e-3  Rs=1e5  Cs=inf  Measurements=on
  Scope : Scope
  Scope2 : Scope
  Voltage Measurement : powerlib/Measurements/Voltage Measurement  PhasorSimulation=off  OutputType=Complex  PSBequivalent=0
  a : PMIOPort  Side=Right
  b : PMIOPort  Port=2  Side=Right
  c : PMIOPort  Port=3  Side=Right
  wires:
  S1/1 -> IGBT/Diode/1
  S2/1 -> IGBT/Diode1/1
  S3/1 -> IGBT/Diode2/1
  S4/1 -> IGBT/Diode3/1
  S5/1 -> IGBT/Diode4/1
  S6/1 -> IGBT/Diode5/1
  Current Measurement/1 -> Scope/1
  Voltage Measurement/1 -> Scope2/1
  connections:
  IGBT/Diode/LConn1 -- Current Measurement/RConn1 -- IGBT/Diode4/LConn1 -- IGBT/Diode2/LConn1
  IGBT/Diode5/LConn1 -- IGBT/Diode4/RConn1 -- c/RConn1
  IGBT/Diode3/RConn1 -- IGBT/Diode5/RConn1 -- Voltage Measurement/LConn2 -- DC Voltage Source/LConn1 -- IGBT/Diode1/RConn1
  IGBT/Diode2/RConn1 -- IGBT/Diode3/LConn1 -- b/RConn1
  IGBT/Diode1/LConn1 -- a/RConn1 -- IGBT/Diode/RConn1
  Voltage Measurement/LConn1 -- Current Measurement/LConn1 -- DC Voltage Source/RConn1

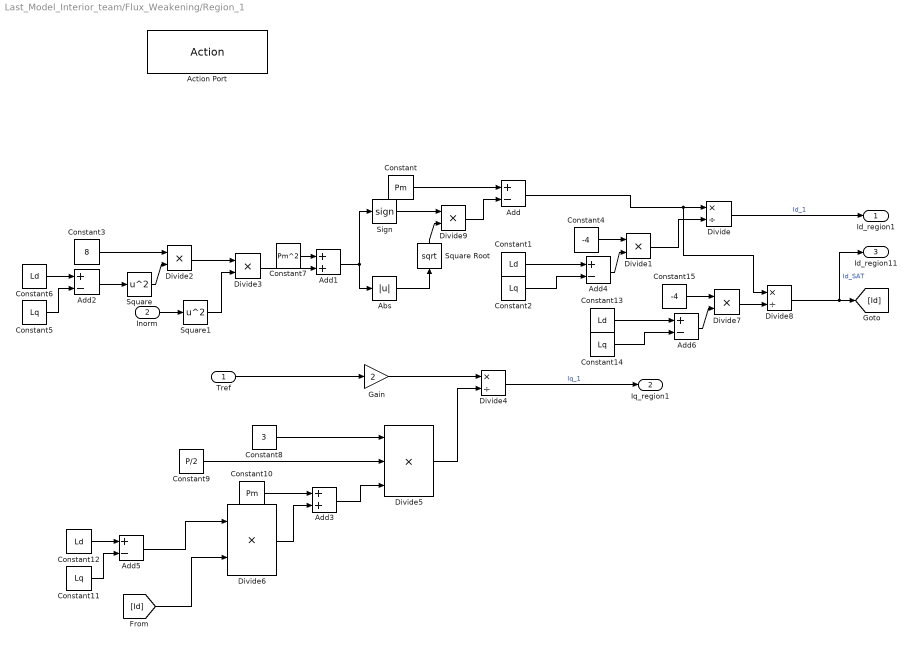
== system Last_Model_Interior_team/Flux_Weakening/Region_1 ==
  Tref : Inport
  Inorm : Inport  Port=2
  Action Port : ActionPort
  Abs : Abs
  Add{,2,4..6} (5 alike) : Sum  Inputs=+-
  Add1 : Sum
  Add3 : Sum
  Constant : Constant  Value=Pm
  Constant{1,6,12..13} (4 alike) : Constant  Value=Ld
  Constant10 : Constant  Value=Pm
  Constant{2,5,11,14} (4 alike) : Constant  Value=Lq
  Constant15 : Constant  Value=-4
  Constant3 : Constant  Value=8
  Constant4 : Constant  Value=-4
  Constant7 : Constant  Value=Pm^2
  Constant8 : Constant  Value=3
  Constant9 : Constant  Value=P/2
  Divide : Product  Inputs=*/
  Divide{1..3,6..7,9} (6 alike) : Product  Inputs=**
  Divide4 : Product  Inputs=*/
  Divide5 : Product  Inputs=***
  Divide8 : Product  Inputs=*/
  Gain : Gain  Gain=2
  Sign : Signum
  Square : Math  Operator=square  SaturateOnIntegerOverflow=on
  Square Root : Sqrt  SaturateOnIntegerOverflow=on
  Square1 : Math  Operator=square  SaturateOnIntegerOverflow=on
  Id_region1 : Outport  InitialOutput=[0]
  Iq_region1 : Outport  Port=2
  Id_region11 : Outport  Port=3  InitialOutput=[0]
  wires:
  Divide/1 -> Id_region1/1  "Id_1"
  Constant/1 -> Add/1
  Constant3/1 -> Divide2/1
  Add2/1 -> Square/1
  Constant5/1 -> Add2/2
  Constant6/1 -> Add2/1
  Square/1 -> Divide2/2
  Inorm/1 -> Square1/1
  Divide2/1 -> Divide3/1
  Square1/1 -> Divide3/2
  Abs/1 -> Square Root/1
  Add/1 -> Divide8/1, Divide/1
  Constant4/1 -> Divide1/1
  Constant1/1 -> Add4/1
  Constant2/1 -> Add4/2
  Add4/1 -> Divide1/2
  Divide1/1 -> Divide/2
  Divide3/1 -> Add1/2
  Constant7/1 -> Add1/1
  Add1/1 -> Sign/1, Abs/1
  Tref/1 -> Gain/1
  Gain/1 -> Divide4/1
  Constant8/1 -> Divide5/1
  Constant9/1 -> Divide5/2
  Constant10/1 -> Add3/1
  Constant12/1 -> Add5/1
  Constant11/1 -> Add5/2
  Add5/1 -> Divide6/1
  [Id] -> Divide6/2
  Divide6/1 -> Add3/2
  Add3/1 -> Divide5/3
  Divide5/1 -> Divide4/2
  Divide4/1 -> Iq_region1/1  "Iq_1"
  Add6/1 -> Divide7/2
  Constant14/1 -> Add6/2
  Constant13/1 -> Add6/1
  Constant15/1 -> Divide7/1
  Divide7/1 -> Divide8/2
  Divide8/1 -> Id_region11/1, [Id]  "Id_SAT"
  Square Root/1 -> Divide9/2
  Sign/1 -> Divide9/1
  Divide9/1 -> Add/2

== system Last_Model_Interior_team/Flux_Weakening/Region_2 ==
  Tref : Inport
  we : Inport  Port=2
  Vmax : Inport  Port=3
  In4 : Inport  Port=4
  Action Port : ActionPort
  Add3 : Sum
  Add5 : Sum  Inputs=+-
  Constant : Constant  Value=-500
  Constant1 : Constant  Value=-500
  Constant10 : Constant  Value=Pm
  Constant11 : Constant  Value=Lq
  Constant12 : Constant  Value=Ld
  Constant8 : Constant  Value=3
  Constant9 : Constant  Value=P/2
  Divide4 : Product  Inputs=*/
  Divide5 : Product  Inputs=***
  Divide6 : Product  Inputs=**
  Gain : Gain  Gain=2
  Saturation Dynamic : simulink/Discontinuities/Saturation Dynamic  OutMin=[]  OutMax=[]  OutDataTypeStr=Inherit: Same as second input  OutDataType=fixdt(1, 16)  OutScaling=2^-10  DoSatur=off
  Saturation Dynamic1 : simulink/Discontinuities/Saturation Dynamic  OutMin=[]  OutMax=[]  OutDataTypeStr=Inherit: Same as second input  OutDataType=fixdt(1, 16)  OutScaling=2^-10  DoSatur=off
  Subsystem : Subsystem
  Id_region2 : Outport
  Iq_region2 : Outport  Port=2
  wires:
  we/1 -> Subsystem/1(we)
  Vmax/1 -> Subsystem/3(Vmax)
  Subsystem/1(Id) -> Saturation Dynamic1/2, Saturation Dynamic/2
  Gain/1 -> Divide4/1
  Divide6/1 -> Add3/2
  Constant10/1 -> Add3/1
  Add5/1 -> Divide6/1
  Divide4/1 -> Iq_region2/1  "Iq_2"
  Add3/1 -> Divide5/3
  Constant9/1 -> Divide5/2
  Constant11/1 -> Add5/2
  Divide5/1 -> Divide4/2
  Constant8/1 -> Divide5/1
  Constant12/1 -> Add5/1
  [Id] -> Divide6/2
  Tref/1 -> Gain/1, Subsystem/2(Tref)
  Constant/1 -> Saturation Dynamic/3
  Saturation Dynamic/1 -> Id_region2/1  "Id_2"
  Constant1/1 -> Saturation Dynamic1/3
  In4/1 -> Saturation Dynamic1/1, Saturation Dynamic/1
  Saturation Dynamic1/1 -> [Id]  "Id_2"

== system Last_Model_Interior_team/Flux_Weakening/Region_3 ==
  We : Inport
  Vmax : Inport  Port=2
  Tref : Inport  Port=3
  Action Port : ActionPort
  Abs : Abs
  Add : Sum  Inputs=+-
  Add3 : Sum
  Add5 : Sum  Inputs=+-
  Constant : Constant  Value=I_Limit
  Constant10 : Constant  Value=Pm
  Constant11 : Constant  Value=Lq
  Constant12 : Constant  Value=Ld
  Constant8 : Constant  Value=3
  Constant9 : Constant  Value=P/2
  Divide4 : Product  Inputs=*/
  Divide5 : Product  Inputs=***
  Divide6 : Product  Inputs=**
  Gain : Gain  Gain=2
  Math Function1 : Math  Operator=magnitude^2  OutputSignalType=real  SaturateOnIntegerOverflow=on
  Math Function2 : Math  Operator=magnitude^2  OutputSignalType=real  SaturateOnIntegerOverflow=on
  Relational Operator : RelationalOperator  Operator=<=  OutDataTypeStr=boolean  RndMeth=Simplest
  Saturation : Saturate  UpperLimit=400  LowerLimit=-400
  Saturation1 : Saturate  UpperLimit=400  LowerLimit=-400
  Scope : Scope
  Sqrt : Sqrt  OutputSignalType=real  SaturateOnIntegerOverflow=on
  Subsystem1 : Subsystem
  Switch : Switch  Criteria=u2 > Threshold
  Id : Outport
  iq : Outport  Port=2
  wires:
  We/1 -> Subsystem1/1(We)
  Constant/1 -> Math Function2/1
  Math Function2/1 -> Add/1
  Math Function1/1 -> Add/2
  Add/1 -> Abs/1
  Sqrt/1 -> Switch/3, Relational Operator/2  "Iq_3"
  Vmax/1 -> Subsystem1/2(Vmax)
  Subsystem1/1(Id) -> [Id], Scope/1, Saturation1/1, Saturation/1  "Id_3"
  Abs/1 -> Sqrt/1
  Saturation/1 -> Math Function1/1
  Saturation1/1 -> Id/1  "Id_3"
  Divide6/1 -> Add3/2
  [Id] -> Divide6/2
  Add5/1 -> Divide6/1
  Constant8/1 -> Divide5/1
  Gain/1 -> Divide4/1
  Divide5/1 -> Divide4/2
  Constant12/1 -> Add5/1
  Constant10/1 -> Add3/1
  Add3/1 -> Divide5/3
  Constant9/1 -> Divide5/2
  Tref/1 -> Gain/1
  Constant11/1 -> Add5/2
  Divide4/1 -> Switch/1, Relational Operator/1  "Iq_3"
  Switch/1 -> iq/1  "Iq_3"
  Relational Operator/1 -> Switch/2

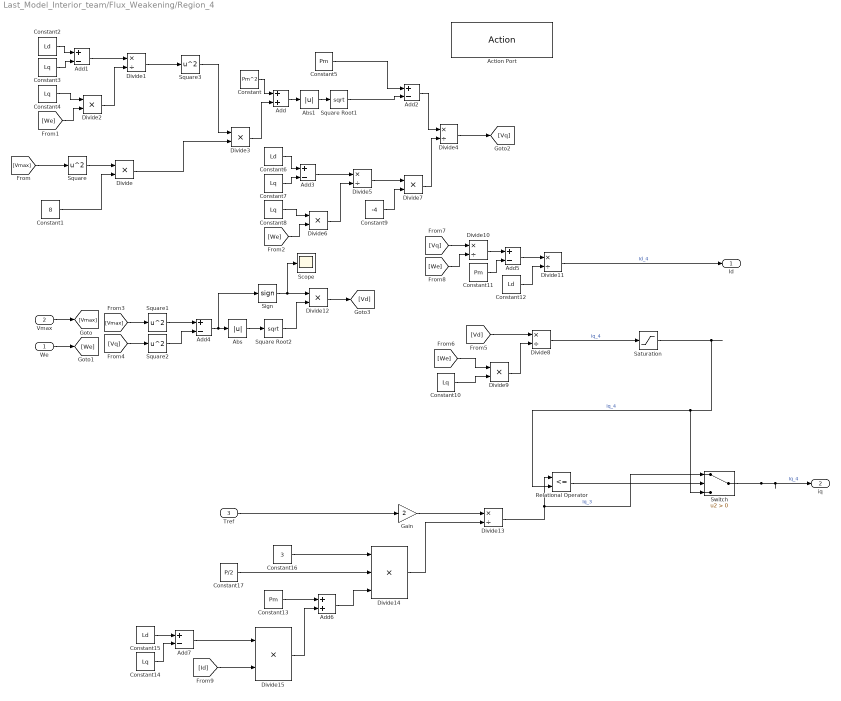
== system Last_Model_Interior_team/Flux_Weakening/Region_4 ==
  We : Inport
  Vmax : Inport  Port=2
  Tref : Inport  Port=3
  Action Port : ActionPort
  Abs : Abs
  Abs1 : Abs
  Add : Sum
  Add{1..5,7} (6 alike) : Sum  Inputs=+-
  Add6 : Sum
  Constant : Constant  Value=Pm^2
  Constant1 : Constant  Value=8
  Constant{3..4,7..8,10,14} (6 alike) : Constant  Value=Lq
  Constant11 : Constant  Value=Pm
  Constant{2,6,12,15} (4 alike) : Constant  Value=Ld
  Constant13 : Constant  Value=Pm
  Constant16 : Constant  Value=3
  Constant17 : Constant  Value=P/2
  Constant5 : Constant  Value=Pm
  Constant9 : Constant  Value=-4
  Divide{,2..3,6..7,9,12,15} (8 alike) : Product  Inputs=**
  Divide{1,4..5,8,10..11,13} (7 alike) : Product  Inputs=*/
  Divide14 : Product  Inputs=***
  Gain : Gain  Gain=2
  Relational Operator : RelationalOperator  Operator=<=  OutDataTypeStr=boolean  RndMeth=Simplest
  Saturation : Saturate  UpperLimit=500  LowerLimit=0
  Scope : Scope
  Sign : Signum
  Square{,1..3} (4 alike) : Math  Operator=square  SaturateOnIntegerOverflow=on
  Square Root1 : Sqrt  OutputSignalType=real  SaturateOnIntegerOverflow=on
  Square Root2 : Sqrt  OutputSignalType=real  SaturateOnIntegerOverflow=on
  Switch : Switch  Criteria=u2 > Threshold
  Id : Outport
  iq : Outport  Port=2
  wires:
  Divide8/1 -> Saturation/1  "Iq_4"
  Divide11/1 -> Id/1  "Id_4"
  Constant/1 -> Add/1
  Vmax/1 -> [Vmax]
  We/1 -> [We]
  [Vmax] -> Square/1
  Square/1 -> Divide/1
  Constant1/1 -> Divide/2
  Constant2/1 -> Add1/1
  Constant3/1 -> Add1/2
  Add1/1 -> Divide1/1
  Constant4/1 -> Divide2/1
  [We] -> Divide2/2
  Divide2/1 -> Divide1/2
  Divide1/1 -> Square3/1
  Divide/1 -> Divide3/2
  Divide3/1 -> Add/2
  Constant5/1 -> Add2/1
  Add2/1 -> Divide4/1
  Divide5/1 -> Divide7/1
  Divide6/1 -> Divide5/2
  [We] -> Divide6/2
  Constant8/1 -> Divide6/1
  Add3/1 -> Divide5/1
  Constant7/1 -> Add3/2
  Constant6/1 -> Add3/1
  Constant9/1 -> Divide7/2
  Divide7/1 -> Divide4/2
  Divide4/1 -> [Vq]
  [Vmax] -> Square1/1
  Square1/1 -> Add4/1
  [Vq] -> Square2/1
  Square2/1 -> Add4/2
  [Vd] -> Divide8/1
  [We] -> Divide9/1
  Constant10/1 -> Divide9/2
  Divide9/1 -> Divide8/2
  [Vq] -> Divide10/1
  [We] -> Divide10/2
  Divide10/1 -> Add5/1
  Constant11/1 -> Add5/2
  Add5/1 -> Divide11/1
  Constant12/1 -> Divide11/2
  Square3/1 -> Divide3/1
  Add4/1 -> Sign/1, Abs/1
  Abs/1 -> Square Root2/1
  Sign/1 -> Divide12/1, Scope/1
  Square Root2/1 -> Divide12/2
  Divide12/1 -> [Vd]
  Add/1 -> Abs1/1
  Abs1/1 -> Square Root1/1
  Square Root1/1 -> Add2/2
  Saturation/1 -> Relational Operator/2, Switch/3  "Iq_4"
  Divide14/1 -> Divide13/2
  Constant15/1 -> Add7/1
  Constant16/1 -> Divide14/1
  Gain/1 -> Divide13/1
  Divide15/1 -> Add6/2
  Add7/1 -> Divide15/1
  [Id] -> Divide15/2
  Tref/1 -> Gain/1
  Constant17/1 -> Divide14/2
  Add6/1 -> Divide14/3
  Constant13/1 -> Add6/1
  Constant14/1 -> Add7/2
  Divide13/1 -> Switch/1, Relational Operator/1  "Iq_3"
  Relational Operator/1 -> Switch/2
  Switch/1 -> iq/1  "Iq_4"

== system Last_Model_Interior_team/Flux_Weakening/Saturation limits ==
  Id_unsat : Inport
  Iq_unsat : Inport  Port=2
  Abs : Abs
  Abs1 : Abs
  Add : Sum
  Constant : Constant  Value=I_Limit
  Constant2 : Constant  Value=I_Limit
  Divide : Product  Inputs=**/
  Divide1 : Product  Inputs=**/
  Math Function : Math  Operator=magnitude^2  SaturateOnIntegerOverflow=on
  Math Function1 : Math  Operator=magnitude^2  SaturateOnIntegerOverflow=on
  Multiply : Gain  Gain=-1
  Multiply1 : Gain  Gain=-1
  Saturation Dynamic : simulink/Discontinuities/Saturation Dynamic  OutMin=[]  OutMax=[]  OutDataTypeStr=Inherit: Same as second input  OutDataType=fixdt(1, 16)  OutScaling=2^-10  DoSatur=off
  Saturation Dynamic1 : simulink/Discontinuities/Saturation Dynamic  OutMin=[]  OutMax=[]  OutDataTypeStr=Inherit: Same as second input  OutDataType=fixdt(1, 16)  OutScaling=2^-10  DoSatur=off
  Sqrt : Sqrt  SaturateOnIntegerOverflow=on
  Zero detection : Subsystem
  Id_Saturated : Outport
  Iq_Saturated : Outport  Port=2
  wires:
  Id_unsat/1 -> Abs1/1, Math Function1/1, [Vd_unsat]
  Math Function/1 -> Add/1
  Math Function1/1 -> Add/2
  Add/1 -> Sqrt/1
  Sqrt/1 -> Zero detection/1(In1)
  Zero detection/1(Out1) -> Divide1/3, Divide/3  "Vs_unsat"
  Iq_unsat/1 -> [Vq_unsat], Abs/1, Math Function/1
  Abs/1 -> Divide/2
  Constant/1 -> Divide/1
  Constant2/1 -> Divide1/1
  Abs1/1 -> Divide1/2
  Divide/1 -> Saturation Dynamic/1, Multiply/1
  [Vq_unsat] -> Saturation Dynamic/2
  Multiply/1 -> Saturation Dynamic/3
  [Vd_unsat] -> Saturation Dynamic1/2
  Divide1/1 -> Multiply1/1, Saturation Dynamic1/1
  Multiply1/1 -> Saturation Dynamic1/3
  Saturation Dynamic/1 -> Iq_Saturated/1
  Saturation Dynamic1/1 -> Id_Saturated/1

== system Last_Model_Interior_team/Flux_Weakening/Subsystem1 ==
  We : Inport
  Id : Inport  Port=2
  Iq : Inport  Port=3
  Add : Sum
  Add1 : Sum
  Constant : Constant  Value=Lq
  Constant1 : Constant  Value=Ld
  Constant2 : Constant  Value=Pm
  Divide : Product  Inputs=***
  Divide1 : Product  Inputs=***
  Divide2 : Product  Inputs=**
  Math Function1 : Math  Operator=magnitude^2  OutputSignalType=real  SaturateOnIntegerOverflow=on
  Math Function2 : Math  Operator=magnitude^2  OutputSignalType=real  SaturateOnIntegerOverflow=on
  Sqrt : Sqrt  OutputSignalType=real  SaturateOnIntegerOverflow=on
  Vmax : Outport
  wires:
  We/1 -> Divide/1, [We]
  Id/1 -> Divide1/1
  Iq/1 -> Divide/2
  Constant/1 -> Divide/3
  Divide/1 -> Math Function1/1
  Math Function1/1 -> Add/1
  [We] -> Divide1/2
  Constant1/1 -> Divide1/3
  Divide1/1 -> Add1/1
  [We] -> Divide2/1
  Constant2/1 -> Divide2/2
  Divide2/1 -> Add1/2
  Add1/1 -> Math Function2/1
  Math Function2/1 -> Add/2
  Add/1 -> Sqrt/1
  Sqrt/1 -> Vmax/1

== system Last_Model_Interior_team/Pi controller D phase/Pi D Phase ==
  Id* : Inport
  Add : Sum
  Discrete-Time Integrator : DiscreteIntegrator  InitialConditionSetting=State (most efficient)  SampleTime=-1  ICPrevOutput=DiscIntNeverNeededParam  ICPrevScaledInput=DiscIntNeverNeededParam
  Gain1 : Gain  Gain=Kp_d*Ki_d
  Gain2 : Gain  Gain=Kp_d
  Vd : Outport
  wires:
  Gain1/1 -> Discrete-Time Integrator/1
  Gain2/1 -> Add/1
  Add/1 -> Vd/1
  Discrete-Time Integrator/1 -> Add/2
  Id*/1 -> Gain2/1, Gain1/1

== system Last_Model_Interior_team/Pi controller Q phase/PI controller ==
  Iq* : Inport
  Add : Sum
  Discrete-Time Integrator : DiscreteIntegrator  InitialConditionSetting=State (most efficient)  SampleTime=-1  ICPrevOutput=DiscIntNeverNeededParam  ICPrevScaledInput=DiscIntNeverNeededParam
  Gain1 : Gain  Gain=Kp_q*Ki_q
  Gain2 : Gain  Gain=Kp_q
  Vq : Outport
  wires:
  Iq*/1 -> Gain1/1, Gain2/1
  Discrete-Time Integrator/1 -> Add/2
  Add/1 -> Vq/1
  Gain2/1 -> Add/1
  Gain1/1 -> Discrete-Time Integrator/1

== system Last_Model_Interior_team/Saturation limits/Zero detection ==
  In1 : Inport
  Constant : Constant  Value=eps
  Switch : Switch  Criteria=u2 > Threshold  Threshold=eps
  Out1 : Outport
  wires:
  Switch/1 -> Out1/1
  Constant/1 -> Switch/3
  In1/1 -> Switch/2, Switch/1

== system Last_Model_Interior_team/Speed Loop/speed_controller ==
  ref_speed : Inport
  Add : Sum
  Discrete-Time Integrator : DiscreteIntegrator  InitialConditionSetting=State (most efficient)  SampleTime=-1  ICPrevOutput=DiscIntNeverNeededParam  ICPrevScaledInput=DiscIntNeverNeededParam
  Gain1 : Gain  Gain=Kp_Speed*Ki_Speed
  Gain2 : Gain  Gain=Kp_Speed
  Saturation : Saturate  UpperLimit=Tfl  LowerLimit=-Tfl
  T_ref : Outport
  wires:
  ref_speed/1 -> Gain1/1, Gain2/1
  Discrete-Time Integrator/1 -> Add/2
  Add/1 -> Saturation/1
  Gain2/1 -> Add/1
  Gain1/1 -> Discrete-Time Integrator/1
  Saturation/1 -> T_ref/1

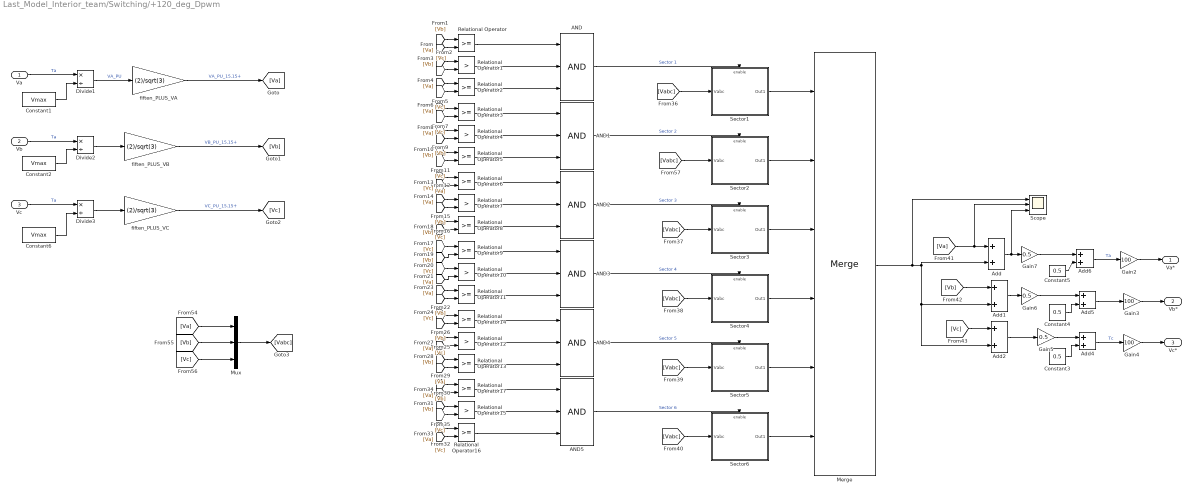
== system Last_Model_Interior_team/Switching/+120_deg_Dpwm ==
  Va : Inport
  Vb : Inport  Port=2
  Vc : Inport  Port=3
  AND{,1..5} (6 alike) : Logic  Inputs=3  IconShape=distinctive  AllPortsSameDT=off  OutDataTypeStr=boolean
  Add{,1..2,4..6} (6 alike) : Sum
  Constant1 : Constant  Value=Vmax
  Constant2 : Constant  Value=Vmax
  Constant3 : Constant  Value=0.5
  Constant4 : Constant  Value=0.5
  Constant5 : Constant  Value=0.5
  Constant6 : Constant  Value=Vmax
  Divide1 : Product  Inputs=*/
  Divide2 : Product  Inputs=*/
  Divide3 : Product  Inputs=*/
  Gain2 : Gain  Gain=100
  Gain3 : Gain  Gain=100
  Gain4 : Gain  Gain=100
  Gain5 : Gain  Gain=0.5
  Gain6 : Gain  Gain=0.5
  Gain7 : Gain  Gain=0.5
  Merge : Merge  Inputs=6
  Mux : Mux  Inputs=3
  Relational Operator{,2..3,5..6,8..9,11,13..14,16..17} (12 alike) : RelationalOperator  OutDataTypeStr=boolean  RndMeth=Simplest
  Relational Operator{1,4,7,10,12,15} (6 alike) : RelationalOperator  Operator=>  OutDataTypeStr=boolean  RndMeth=Simplest
  Scope : Scope  NumInputPorts=3
  Sector1 : Subsystem  TreatAsAtomicUnit=on
  Sector2 : Subsystem  TreatAsAtomicUnit=on
  Sector3 : Subsystem  TreatAsAtomicUnit=on
  Sector4 : Subsystem  TreatAsAtomicUnit=on
  Sector5 : Subsystem  TreatAsAtomicUnit=on
  Sector6 : Subsystem  TreatAsAtomicUnit=on
  fiften_PLUS_VA : Gain  Gain=(2)/sqrt(3)  RndMeth=Simplest  OutDataTypeStr=Inherit: Same as input  ParamDataTypeStr=Inherit: Same as input
  fiften_PLUS_VB : Gain  Gain=(2)/sqrt(3)  RndMeth=Simplest  OutDataTypeStr=Inherit: Same as input  ParamDataTypeStr=Inherit: Same as input
  fiften_PLUS_VC : Gain  Gain=(2)/sqrt(3)  RndMeth=Simplest  OutDataTypeStr=Inherit: Same as input  ParamDataTypeStr=Inherit: Same as input
  Va* : Outport
  Vb* : Outport  Port=2
  Vc* : Outport  Port=3
  wires:
  Add/1 -> Gain7/1, Scope/3
  Merge/1 -> Add1/2, Add2/2, Add/2, Scope/1
  Mux/1 -> [Vabc]
  Add6/1 -> Gain2/1  "Ta"
  Add4/1 -> Gain4/1  "Tc"
  Add5/1 -> Gain3/1
  Add2/1 -> Gain5/1
  Constant5/1 -> Add6/2
  Gain7/1 -> Add6/1
  Constant4/1 -> Add5/2
  Constant3/1 -> Add4/2
  Gain5/1 -> Add4/1
  [Vb] -> Add1/1
  [Vc] -> Add2/1
  Sector4/1(Out1) -> Merge/4
  Sector5/1(Out1) -> Merge/5
  Sector3/1(Out1) -> Merge/3
  [Vabc] -> Sector3/1(Vabc)
  Sector6/1(Out1) -> Merge/6
  Sector2/1(Out1) -> Merge/2
  [Va] -> Relational Operator10/2
  [Vb] -> Relational Operator8/2
  [Va] -> Relational Operator13/2
  [Va] -> Relational Operator7/1
  Gain3/1 -> Vb*/1
  [Va] -> Relational Operator6/1
  [Vc] -> Relational Operator6/2
  [Vb] -> Relational Operator7/2
  [Vb] -> Relational Operator9/2
  [Vb] -> Relational Operator14/2
  [Vc] -> Relational Operator16/1
  [Vabc] -> Sector2/1(Vabc)
  [Vc] -> Relational Operator8/1
  [Vc] -> Relational Operator1/2
  Relational Operator8/1 -> AND2/3
  Relational Operator6/1 -> AND2/1
  Relational Operator4/1 -> AND1/2
  Relational Operator5/1 -> AND1/3
  [Vb] -> Relational Operator5/1
  Add1/1 -> Gain6/1
  Relational Operator10/1 -> AND3/2
  [Vabc] -> Sector1/1(Vabc)
  [Vc] -> Relational Operator9/1
  Relational Operator14/1 -> AND4/1
  Relational Operator13/1 -> AND4/3
  [Vc] -> Relational Operator10/1
  [Vc] -> Relational Operator14/1
  [Vb] -> Mux/2
  [Vc] -> Relational Operator3/2
  Relational Operator2/1 -> AND/3
  [Vc] -> Relational Operator15/2
  [Vabc] -> Sector6/1(Vabc)
  Relational Operator7/1 -> AND2/2
  [Vc] -> Relational Operator12/1
  [Va] -> Mux/1
  [Va] -> Relational Operator11/1
  Relational Operator9/1 -> AND3/1
  Relational Operator1/1 -> AND/2
  Gain2/1 -> Va*/1
  [Vb] -> Relational Operator17/1
  Gain6/1 -> Add5/1
  [Vb] -> Relational Operator4/2
  [Vb] -> Relational Operator1/1
  Gain4/1 -> Vc*/1
  Sector1/1(Out1) -> Merge/1
  [Vc] -> Mux/3
  Relational Operator3/1 -> AND1/1
  Relational Operator/1 -> AND/1
  [Va] -> Relational Operator/2
  [Va] -> Relational Operator3/1
  Relational Operator12/1 -> AND4/2
  Relational Operator15/1 -> AND5/2
  [Va] -> Relational Operator17/2
  Relational Operator16/1 -> AND5/3
  [Vc] -> Relational Operator2/2
  [Vb] -> Relational Operator15/1
  Relational Operator11/1 -> AND3/3
  [Va] -> Add/1, Scope/2
  [Vabc] -> Sector5/1(Vabc)
  [Vb] -> Relational Operator/1
  [Vc] -> Relational Operator5/2
  [Vb] -> Relational Operator13/1
  [Va] -> Relational Operator16/2
  [Vabc] -> Sector4/1(Vabc)
  [Va] -> Relational Operator12/2
  Relational Operator17/1 -> AND5/1
  [Vb] -> Relational Operator11/2
  [Va] -> Relational Operator2/1
  [Va] -> Relational Operator4/1
  AND/1 -> Sector1/Enable  "Sector 1"
  AND1/1 -> Sector2/Enable  "Sector 2"
  AND2/1 -> Sector3/Enable  "Sector 3"
  AND3/1 -> Sector4/Enable  "Sector 4"
  AND4/1 -> Sector5/Enable  "Sector 5"
  AND5/1 -> Sector6/Enable  "Sector 6"
  Constant2/1 -> Divide2/2
  Vc/1 -> Divide3/1  "Ta"
  Divide1/1 -> fiften_PLUS_VA/1  "VA_PU"
  Divide3/1 -> fiften_PLUS_VC/1
  fiften_PLUS_VA/1 -> [Va]  "VA_PU_15.15+"
  Vb/1 -> Divide2/1  "Ta"
  Constant1/1 -> Divide1/2
  Va/1 -> Divide1/1  "Ta"
  Constant6/1 -> Divide3/2
  Divide2/1 -> fiften_PLUS_VB/1
  fiften_PLUS_VB/1 -> [Vb]  "VB_PU_15.15+"
  fiften_PLUS_VC/1 -> [Vc]  "VC_PU_15.15+"
